simulink library "DBL_MasterLib"  (R2020b)
settings: Solver=VariableStepAuto  StartTime=0.0  StopTime=10.0  RelTol=1e-3
libraries: simulink x5, $bdroot x1
settings Model: Creator=ahashem  LastModifiedBy=ahashem

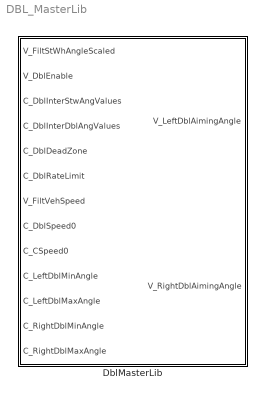
== system DBL_MasterLib ==
  DblMasterLib : Subsystem

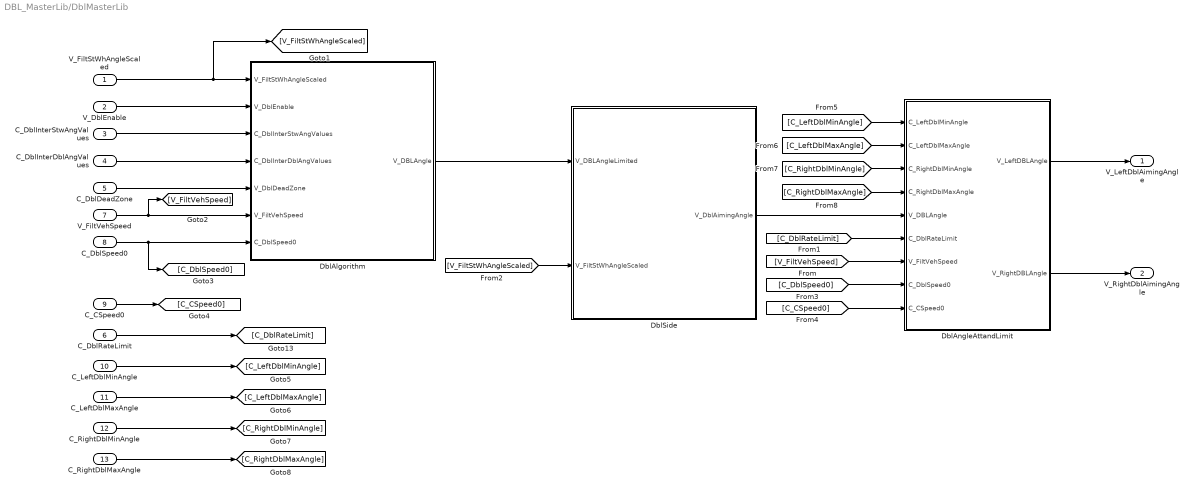
== system DBL_MasterLib/DblMasterLib ==
  V_FiltStWhAngleScaled : Inport  RequirementInfo={} %GIDa_60832143_23e3_4e37_9ef8_f4c8fbc195ea
  V_DblEnable : Inport  Port=2
  C_DblInterStwAngValues : Inport  Port=3
  C_DblInterDblAngValues : Inport  Port=4
  C_DblDeadZone : Inport  Port=5
  C_DblRateLimit : Inport  Port=6
  V_FiltVehSpeed : Inport  Port=7
  C_DblSpeed0 : Inport  Port=8
  C_CSpeed0 : Inport  Port=9
  C_LeftDblMinAngle : Inport  Port=10
  C_LeftDblMaxAngle : Inport  Port=11
  C_RightDblMinAngle : Inport  Port=12
  C_RightDblMaxAngle : Inport  Port=13
  DblAlgorithm : Subsystem  TreatAsAtomicUnit=on
  DblAngleAttandLimit : Subsystem
  DblSide : Subsystem
  V_LeftDblAimingAngle : Outport  RequirementInfo={} %GIDa_20373fde_4aa9_40e5_8d80_7fd2414d965e  VectorParamsAs1DForOutWhenUnconnected=off
  V_RightDblAimingAngle : Outport  Port=2  VectorParamsAs1DForOutWhenUnconnected=off
  wires:
  DblAlgorithm/1(V_DBLAngle) -> DblSide/1(V_DBLAngleLimited)
  DblSide/1(V_DblAimingAngle) -> DblAngleAttandLimit/5(V_DBLAngle)
  C_DblInterStwAngValues/1 -> DblAlgorithm/3(C_DblInterStwAngValues)
  C_DblDeadZone/1 -> DblAlgorithm/5(V_DblDeadZone)
  C_DblInterDblAngValues/1 -> DblAlgorithm/4(C_DblInterDblAngValues)
  V_DblEnable/1 -> DblAlgorithm/2(V_DblEnable)
  C_DblRateLimit/1 -> [C_DblRateLimit]
  V_FiltStWhAngleScaled/1 -> [V_FiltStWhAngleScaled], DblAlgorithm/1(V_FiltStWhAngleScaled)
  [V_FiltStWhAngleScaled] -> DblSide/2(V_FiltStWhAngleScaled)
  [C_DblRateLimit] -> DblAngleAttandLimit/6(C_DblRateLimit)
  C_DblSpeed0/1 -> [C_DblSpeed0], DblAlgorithm/7(C_DblSpeed0)
  V_FiltVehSpeed/1 -> [V_FiltVehSpeed], DblAlgorithm/6(V_FiltVehSpeed)
  C_CSpeed0/1 -> [C_CSpeed0]
  [C_DblSpeed0] -> DblAngleAttandLimit/8(C_DblSpeed0)
  [V_FiltVehSpeed] -> DblAngleAttandLimit/7(V_FiltVehSpeed)
  [C_CSpeed0] -> DblAngleAttandLimit/9(C_CSpeed0)
  C_LeftDblMinAngle/1 -> [C_LeftDblMinAngle]
  C_RightDblMaxAngle/1 -> [C_RightDblMaxAngle]
  C_RightDblMinAngle/1 -> [C_RightDblMinAngle]
  C_LeftDblMaxAngle/1 -> [C_LeftDblMaxAngle]
  [C_LeftDblMinAngle] -> DblAngleAttandLimit/1(C_LeftDblMinAngle)
  [C_LeftDblMaxAngle] -> DblAngleAttandLimit/2(C_LeftDblMaxAngle)
  [C_RightDblMinAngle] -> DblAngleAttandLimit/3(C_RightDblMinAngle)
  [C_RightDblMaxAngle] -> DblAngleAttandLimit/4(C_RightDblMaxAngle)
  DblAngleAttandLimit/1(V_LeftDBLAngle) -> V_LeftDblAimingAngle/1
  DblAngleAttandLimit/2(V_RightDBLAngle) -> V_RightDblAimingAngle/1

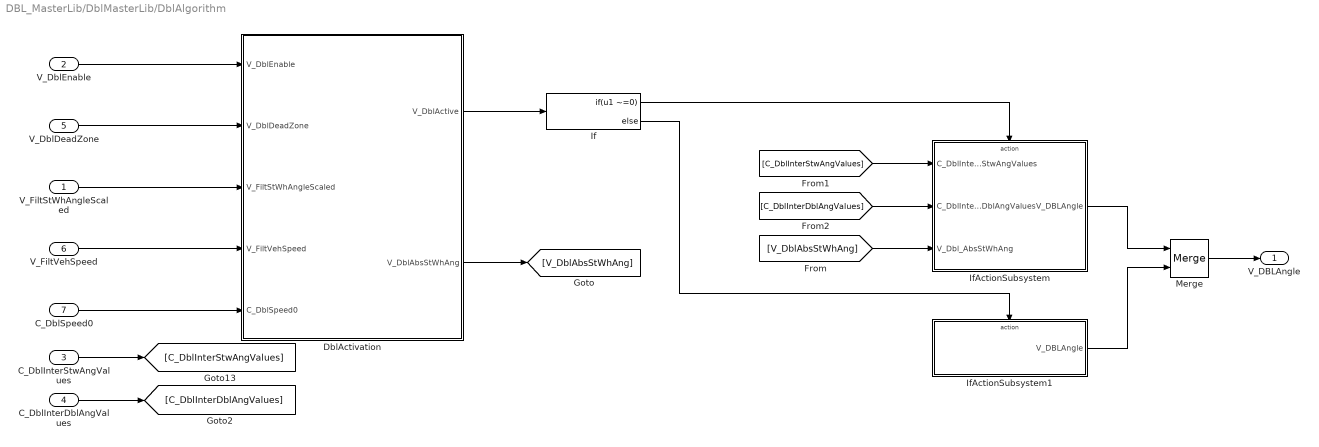
== system DBL_MasterLib/DblMasterLib/DblAlgorithm ==
  V_FiltStWhAngleScaled : Inport
  V_DblEnable : Inport  Port=2
  C_DblInterStwAngValues : Inport  Port=3
  C_DblInterDblAngValues : Inport  Port=4
  V_DblDeadZone : Inport  Port=5
  V_FiltVehSpeed : Inport  Port=6
  C_DblSpeed0 : Inport  Port=7
  DblActivation : Subsystem
  If : If  IfExpression=u1 ~=0
  IfActionSubsystem : Subsystem  TreatAsAtomicUnit=on
  IfActionSubsystem1 : Subsystem  TreatAsAtomicUnit=on
  Merge : Merge
  V_DBLAngle : Outport  VectorParamsAs1DForOutWhenUnconnected=off
  wires:
  C_DblInterStwAngValues/1 -> [C_DblInterStwAngValues]
  Merge/1 -> V_DBLAngle/1
  If/1 -> IfActionSubsystem/Action
  [V_DblAbsStWhAng] -> IfActionSubsystem/3(V_Dbl_AbsStWhAng)
  [C_DblInterStwAngValues] -> IfActionSubsystem/1(C_DblInterStwAngValues)
  If/2 -> IfActionSubsystem1/Action
  IfActionSubsystem/1(V_DBLAngle) -> Merge/1
  IfActionSubsystem1/1(V_DBLAngle) -> Merge/2
  C_DblInterDblAngValues/1 -> [C_DblInterDblAngValues]
  [C_DblInterDblAngValues] -> IfActionSubsystem/2(C_DblInterDblAngValues)
  DblActivation/2(V_DblAbsStWhAng) -> [V_DblAbsStWhAng]
  V_DblEnable/1 -> DblActivation/1(V_DblEnable)
  V_DblDeadZone/1 -> DblActivation/2(V_DblDeadZone)
  V_FiltStWhAngleScaled/1 -> DblActivation/3(V_FiltStWhAngleScaled)
  DblActivation/1(V_DblActive) -> If/1
  V_FiltVehSpeed/1 -> DblActivation/4(V_FiltVehSpeed)
  C_DblSpeed0/1 -> DblActivation/5(C_DblSpeed0)

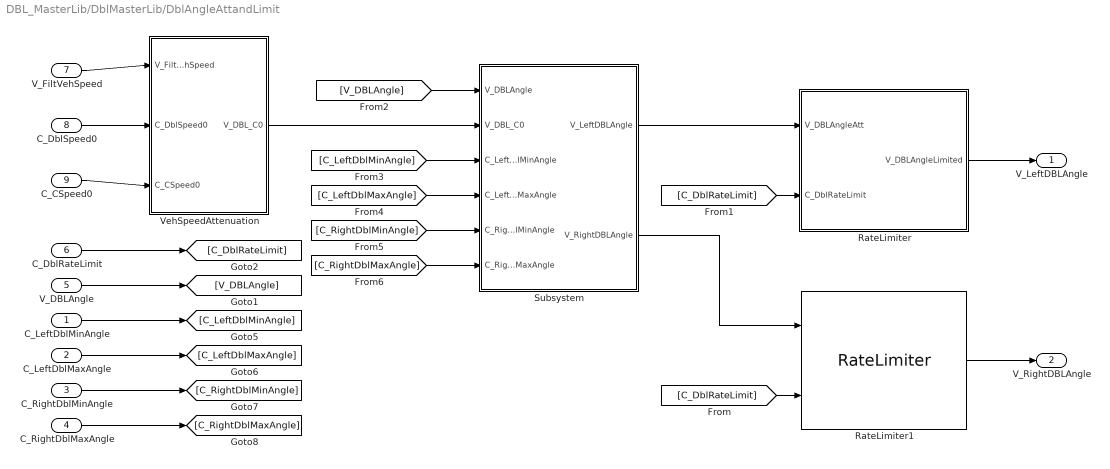
== system DBL_MasterLib/DblMasterLib/DblAngleAttandLimit ==
  C_LeftDblMinAngle : Inport
  C_LeftDblMaxAngle : Inport  Port=2
  C_RightDblMinAngle : Inport  Port=3
  C_RightDblMaxAngle : Inport  Port=4
  V_DBLAngle : Inport  Port=5
  C_DblRateLimit : Inport  Port=6
  V_FiltVehSpeed : Inport  Port=7
  C_DblSpeed0 : Inport  Port=8
  C_CSpeed0 : Inport  Port=9
  RateLimiter : Subsystem
  RateLimiter1 : $bdroot/DblMasterLib/DblAngleAttandLimit/RateLimiter  SystemSampleTime=-1  VariantActivationTime=update diagram  Latency=0  AutoFrameSizeCalculation=off
  Subsystem : Subsystem
  VehSpeedAttenuation : Subsystem
  V_LeftDBLAngle : Outport
  V_RightDBLAngle : Outport  Port=2
  wires:
  V_DBLAngle/1 -> [V_DBLAngle]
  RateLimiter/1(V_DBLAngleLimited) -> V_LeftDBLAngle/1
  V_FiltVehSpeed/1 -> VehSpeedAttenuation/1(V_FiltVehSpeed)
  C_DblSpeed0/1 -> VehSpeedAttenuation/2(C_DblSpeed0)
  C_CSpeed0/1 -> VehSpeedAttenuation/3(C_CSpeed0)
  C_RightDblMaxAngle/1 -> [C_RightDblMaxAngle]
  C_LeftDblMinAngle/1 -> [C_LeftDblMinAngle]
  C_RightDblMinAngle/1 -> [C_RightDblMinAngle]
  C_LeftDblMaxAngle/1 -> [C_LeftDblMaxAngle]
  C_DblRateLimit/1 -> [C_DblRateLimit]
  [C_DblRateLimit] -> RateLimiter1/2
  [C_DblRateLimit] -> RateLimiter/2(C_DblRateLimit)
  RateLimiter1/1 -> V_RightDBLAngle/1
  [V_DBLAngle] -> Subsystem/1(V_DBLAngle)
  VehSpeedAttenuation/1(V_DBL_C0) -> Subsystem/2(V_DBL_C0)
  [C_LeftDblMinAngle] -> Subsystem/3(C_LeftDblMinAngle)
  [C_LeftDblMaxAngle] -> Subsystem/4(C_LeftDblMaxAngle)
  [C_RightDblMinAngle] -> Subsystem/5(C_RightDblMinAngle)
  [C_RightDblMaxAngle] -> Subsystem/6(C_RightDblMaxAngle)
  Subsystem/1(V_LeftDBLAngle) -> RateLimiter/1(V_DBLAngleAtt)
  Subsystem/2(V_RightDBLAngle) -> RateLimiter1/1

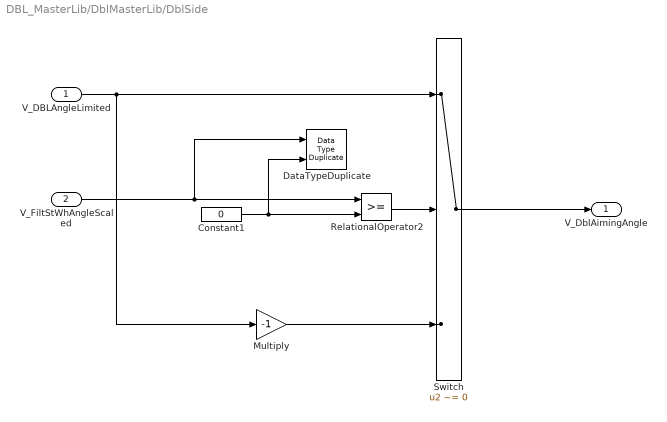
== system DBL_MasterLib/DblMasterLib/DblSide ==
  V_DBLAngleLimited : Inport
  V_FiltStWhAngleScaled : Inport  Port=2
  Constant1 : Constant  Value=0  OutDataTypeStr=Inherit: Inherit via back propagation
  DataTypeDuplicate : DataTypeDuplicate
  Multiply : Gain  Gain=-1  ParamDataTypeStr=int8
  RelationalOperator2 : RelationalOperator  OutDataTypeStr=boolean  RndMeth=Nearest
  Switch : Switch  Criteria=u2 ~= 0  OutDataTypeStr=fixdt(1,16,0.1,0)  RndMeth=Nearest
  V_DblAimingAngle : Outport  VectorParamsAs1DForOutWhenUnconnected=off
  wires:
  RelationalOperator2/1 -> Switch/2
  Switch/1 -> V_DblAimingAngle/1
  V_FiltStWhAngleScaled/1 -> DataTypeDuplicate/1, RelationalOperator2/1
  Constant1/1 -> DataTypeDuplicate/2, RelationalOperator2/2
  V_DBLAngleLimited/1 -> Switch/1, Multiply/1
  Multiply/1 -> Switch/3

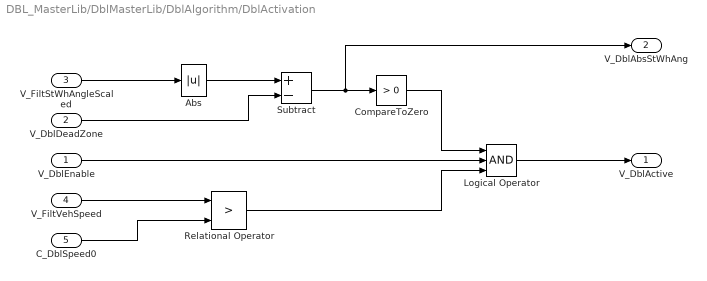
== system DBL_MasterLib/DblMasterLib/DblAlgorithm/DblActivation ==
  V_DblEnable : Inport
  V_DblDeadZone : Inport  Port=2
  V_FiltStWhAngleScaled : Inport  Port=3
  V_FiltVehSpeed : Inport  Port=4
  C_DblSpeed0 : Inport  Port=5
  Abs : Abs  RndMeth=Simplest  SaturateOnIntegerOverflow=on
  CompareToZero : simulink/Logic and Bit Operations/Compare To Zero  relop=>  OutDataTypeStr=boolean
  Logical Operator : Logic  Inputs=3  AllPortsSameDT=off  OutDataTypeStr=boolean
  Relational Operator : RelationalOperator  Operator=>  OutDataTypeStr=boolean  RndMeth=Simplest
  Subtract : Sum  Inputs=+-  OutDataTypeStr=Inherit: Same as first input
  V_DblActive : Outport  VectorParamsAs1DForOutWhenUnconnected=off
  V_DblAbsStWhAng : Outport  Port=2  VectorParamsAs1DForOutWhenUnconnected=off
  wires:
  Logical Operator/1 -> V_DblActive/1
  Abs/1 -> Subtract/1
  Subtract/1 -> CompareToZero/1, V_DblAbsStWhAng/1
  V_DblEnable/1 -> Logical Operator/2
  CompareToZero/1 -> Logical Operator/1
  V_DblDeadZone/1 -> Subtract/2
  V_FiltStWhAngleScaled/1 -> Abs/1
  V_FiltVehSpeed/1 -> Relational Operator/1
  C_DblSpeed0/1 -> Relational Operator/2
  Relational Operator/1 -> Logical Operator/3

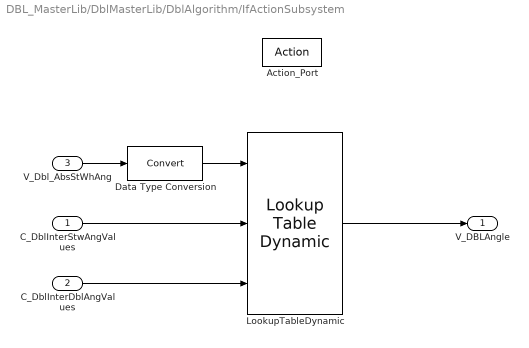
== system DBL_MasterLib/DblMasterLib/DblAlgorithm/IfActionSubsystem ==
  C_DblInterStwAngValues : Inport
  C_DblInterDblAngValues : Inport  Port=2
  V_Dbl_AbsStWhAng : Inport  Port=3
  Action_Port : ActionPort  ActionPortLabel=if(u1 ~=0)
  Data Type Conversion : DataTypeConversion
  LookupTableDynamic : simulink/Lookup Tables/Lookup Table Dynamic  LookUpMeth=Interpolation-Use End Values  OutDataType=fixdt('double')  OutScaling=2^-10  OutDataTypeStr=Inherit: Inherit via back propagation  RndMeth=Simplest  DoSatur=off
  V_DBLAngle : Outport  VectorParamsAs1DForOutWhenUnconnected=off
  wires:
  LookupTableDynamic/1 -> V_DBLAngle/1
  V_Dbl_AbsStWhAng/1 -> Data Type Conversion/1
  C_DblInterStwAngValues/1 -> LookupTableDynamic/2
  C_DblInterDblAngValues/1 -> LookupTableDynamic/3
  Data Type Conversion/1 -> LookupTableDynamic/1

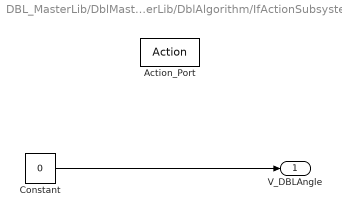
== system DBL_MasterLib/DblMasterLib/DblAlgorithm/IfActionSubsystem1 ==
  Action_Port : ActionPort  ActionPortLabel=else
  Constant : Constant  Value=0  OutDataTypeStr=Inherit: Inherit via back propagation
  V_DBLAngle : Outport
  wires:
  Constant/1 -> V_DBLAngle/1

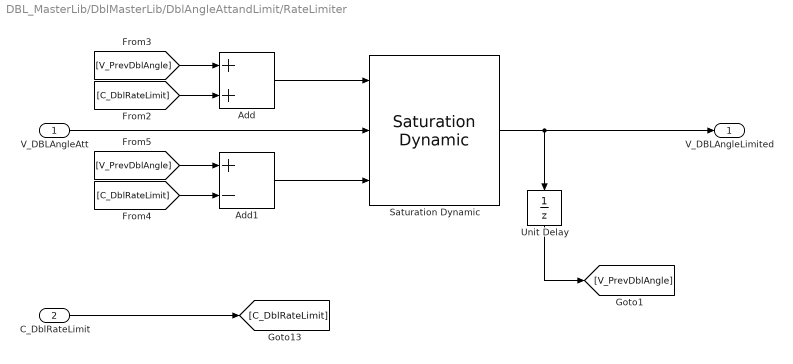
== system DBL_MasterLib/DblMasterLib/DblAngleAttandLimit/RateLimiter ==
  V_DBLAngleAtt : Inport
  C_DblRateLimit : Inport  Port=2
  Add : Sum
  Add1 : Sum  Inputs=+-  AccumDataTypeStr=fixdt(1,16,0.1,0)  OutDataTypeStr=fixdt(1,16,0.1,0)  SaturateOnIntegerOverflow=on
  Saturation Dynamic : simulink/Discontinuities/Saturation Dynamic  OutMin=[]  OutMax=[]  OutDataTypeStr=Inherit: Same as second input  OutDataType=fixdt(1, 16)  OutScaling=2^-10  DoSatur=off
  Unit Delay : UnitDelay  SampleTime=-1  HasFrameUpgradeWarning=on
  V_DBLAngleLimited : Outport
  wires:
  C_DblRateLimit/1 -> [C_DblRateLimit]
  Unit Delay/1 -> [V_PrevDblAngle]
  [C_DblRateLimit] -> Add/2
  Add1/1 -> Saturation Dynamic/3
  [V_PrevDblAngle] -> Add1/1
  Saturation Dynamic/1 -> V_DBLAngleLimited/1, Unit Delay/1
  [V_PrevDblAngle] -> Add/1
  [C_DblRateLimit] -> Add1/2
  Add/1 -> Saturation Dynamic/1
  V_DBLAngleAtt/1 -> Saturation Dynamic/2

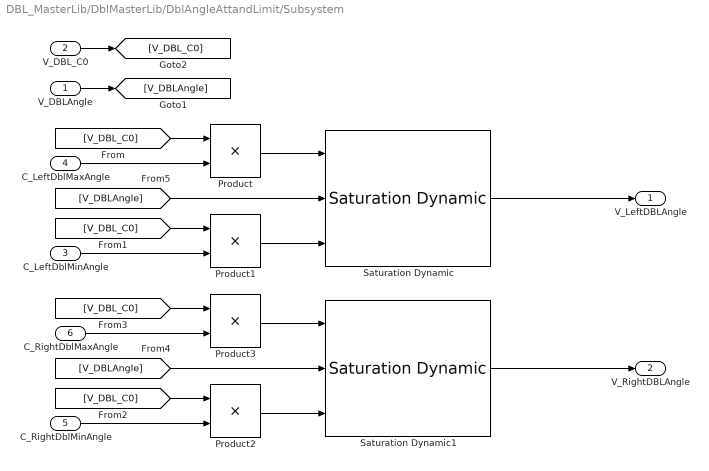
== system DBL_MasterLib/DblMasterLib/DblAngleAttandLimit/Subsystem ==
  V_DBLAngle : Inport
  V_DBL_C0 : Inport  Port=2
  C_LeftDblMinAngle : Inport  Port=3
  C_LeftDblMaxAngle : Inport  Port=4
  C_RightDblMinAngle : Inport  Port=5
  C_RightDblMaxAngle : Inport  Port=6
  Product{,1..3} (4 alike) : Product  RndMeth=Nearest
  Saturation Dynamic : simulink/Discontinuities/Saturation Dynamic  OutMin=[]  OutMax=[]  OutDataTypeStr=Inherit: Same as second input  OutDataType=fixdt(1, 16)  OutScaling=2^-10  RndMeth=Nearest  DoSatur=off
  Saturation Dynamic1 : simulink/Discontinuities/Saturation Dynamic  OutMin=[]  OutMax=[]  OutDataTypeStr=Inherit: Same as second input  OutDataType=fixdt(1, 16)  OutScaling=2^-10  RndMeth=Nearest  DoSatur=off
  V_LeftDBLAngle : Outport
  V_RightDBLAngle : Outport  Port=2
  wires:
  C_LeftDblMaxAngle/1 -> Product/2
  V_DBLAngle/1 -> [V_DBLAngle]
  V_DBL_C0/1 -> [V_DBL_C0]
  [V_DBL_C0] -> Product/1
  Product/1 -> Saturation Dynamic/1
  [V_DBL_C0] -> Product1/1
  C_LeftDblMinAngle/1 -> Product1/2
  Product1/1 -> Saturation Dynamic/3
  C_RightDblMinAngle/1 -> Product2/2
  [V_DBL_C0] -> Product3/1
  Product3/1 -> Saturation Dynamic1/1
  [V_DBL_C0] -> Product2/1
  Product2/1 -> Saturation Dynamic1/3
  C_RightDblMaxAngle/1 -> Product3/2
  [V_DBLAngle] -> Saturation Dynamic1/2
  [V_DBLAngle] -> Saturation Dynamic/2
  Saturation Dynamic/1 -> V_LeftDBLAngle/1
  Saturation Dynamic1/1 -> V_RightDBLAngle/1

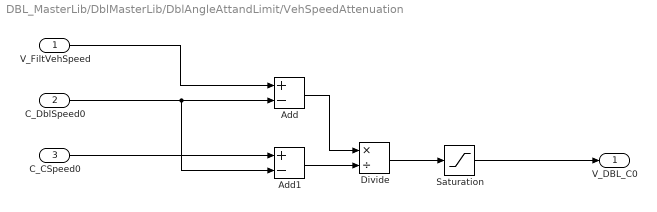
== system DBL_MasterLib/DblMasterLib/DblAngleAttandLimit/VehSpeedAttenuation ==
  V_FiltVehSpeed : Inport
  C_DblSpeed0 : Inport  Port=2
  C_CSpeed0 : Inport  Port=3
  Add : Sum  Inputs=+-  AccumDataTypeStr=fixdt(1,16,0.1,0)  OutDataTypeStr=fixdt(1,16,0.1,0)
  Add1 : Sum  Inputs=+-  AccumDataTypeStr=fixdt(1,16,0.1,0)  OutDataTypeStr=fixdt(1,16,0.1,0)
  Divide : Product  Inputs=*/  OutDataTypeStr=fixdt(1,16,0.01,0)
  Saturation : Saturate  UpperLimit=1  LowerLimit=0
  V_DBL_C0 : Outport
  wires:
  V_FiltVehSpeed/1 -> Add/1
  C_DblSpeed0/1 -> Add1/2, Add/2
  C_CSpeed0/1 -> Add1/1
  Add/1 -> Divide/1
  Add1/1 -> Divide/2
  Divide/1 -> Saturation/1
  Saturation/1 -> V_DBL_C0/1
